simulink library "AEMACE8_INSTRUMENTATION"  (R2021b)
settings: Solver=VariableStepAuto  StartTime=0.0  StopTime=10.0  RelTol=1e-3
undefined symbols (not defined in the file or in its folder): AEMACE8_command, AEMACE8_demand, AEMACE8_demandDCL, AEMACE8_mode, AEMACE8_RLimitedDemand, AEMACE8_RLimitedOffsetFCL
settings Model: Creator=ACH  LastModifiedBy=ACH

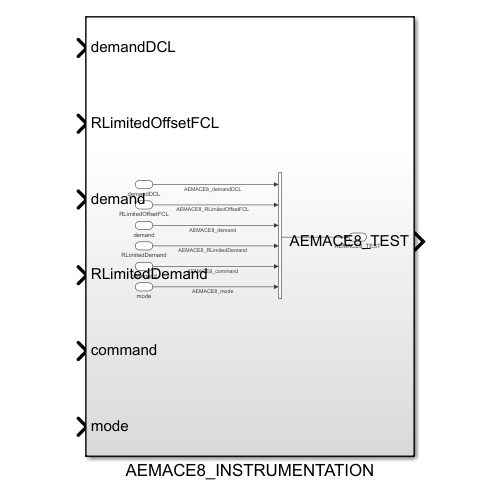
[thumbnail: Simulink's stored preview of the top-level diagram]
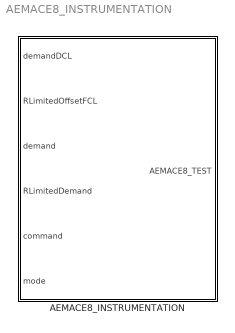
== system AEMACE8_INSTRUMENTATION ==
  AEMACE8_INSTRUMENTATION : Subsystem

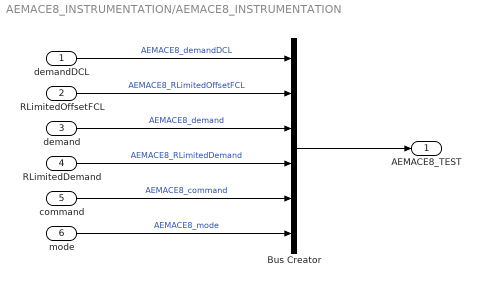
== system AEMACE8_INSTRUMENTATION/AEMACE8_INSTRUMENTATION ==
  demandDCL : Inport
  RLimitedOffsetFCL : Inport  Port=2
  demand : Inport  Port=3
  RLimitedDemand : Inport  Port=4
  command : Inport  Port=5
  mode : Inport  Port=6
  Bus Creator : BusCreator  Inputs=AEMACE8_demandDCL,AEMACE8_RLimitedOffsetFCL,AEMACE8_demand,AEMACE8_RLimitedDemand,AEMACE8_command,AEMACE8_mode  OutDataTypeStr=Bus: AEMACE8_TEST
  AEMACE8_TEST : Outport  OutDataTypeStr=Bus: AEMACE8_TEST
  wires:
  mode/1 -> Bus Creator/6  "AEMACE8_mode"
  demand/1 -> Bus Creator/3  "AEMACE8_demand"
  Bus Creator/1 -> AEMACE8_TEST/1
  command/1 -> Bus Creator/5  "AEMACE8_command"
  demandDCL/1 -> Bus Creator/1  "AEMACE8_demandDCL"
  RLimitedOffsetFCL/1 -> Bus Creator/2  "AEMACE8_RLimitedOffsetFCL"
  RLimitedDemand/1 -> Bus Creator/4  "AEMACE8_RLimitedDemand"
